simulink model "imcpendel4"  (R2021b)
settings: Solver=daessc  StartTime=0.0  StopTime=100  RelTol=1e-3
values from neighbouring files (symbols this model uses):
  A = eval(A)    [pendulum1.m]
  B = eval(B)    [pendulum1.m]
  C = [1 0]    [pendulum1.m]
  D = [0]    [pendulum1.m]
  G_star_filter = G_star_stable*G_filter    [pendulum1.m]
  xR = [pi; 0]    [pendulum1.m]
settings Model: Creator=mluser  LastModifiedBy=1star
settings DebuggingCC: UnconnectedInputMsg=none  UnconnectedOutputMsg=none  UnconnectedLineMsg=none
settings ModelReferenceCC: EnableRefExpFcnMdlSchedulingChecks=off
settings RTWCC: DLArmComputeVersion=20.02.1

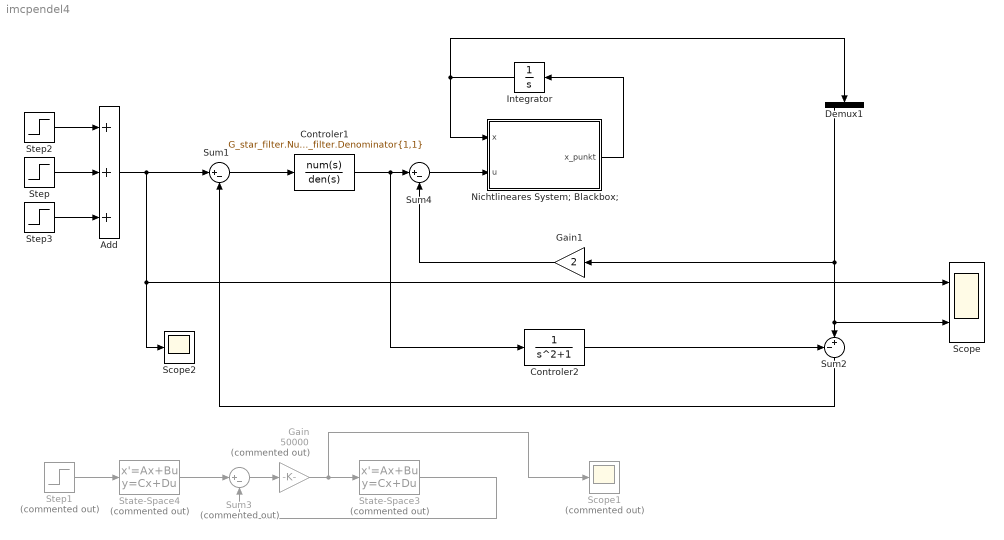
== system imcpendel4 ==
  Add : Sum  Inputs=+++
  Controler1 : TransferFcn  Numerator=G_star_filter.Numerator{1,1}  Denominator=G_star_filter.Denominator{1,1}
  Controler2 : TransferFcn  Numerator=1  Denominator=[1 0 1]
  Demux1 : Demux  Outputs=2
  Gain : Gain  Commented=on  Gain=50000
  Gain1 : Gain  Gain=2
  Integrator : Integrator  InitialCondition=xR
  Nichtlineares System; Blackbox; : MATLAB Function
  Scope : Scope  NumInputPorts=2
  Scope1 : Scope  Commented=on
  Scope2 : Scope
  State-Space3 : StateSpace  Commented=on  A=A  B=B  C=C  D=D  InitialCondition=0
  State-Space4 : StateSpace  Commented=on  A=A  B=B  C=C  D=D  InitialCondition=0
  Step : Step  Time=2  After=0  SampleTime=0
  Step1 : Step  Commented=on  SampleTime=0
  Step2 : Step  Before=pi  After=pi  SampleTime=0
  Step3 : Step  Time=3  After=0  SampleTime=0
  Sum1 : Sum  Inputs=|+-
  Sum2 : Sum  Inputs=-+|
  Sum3 : Sum  Commented=on  Inputs=|+-
  Sum4 : Sum  Inputs=|+-
  wires:
  Controler2/1 -> Sum2/1
  Sum1/1 -> Controler1/1
  State-Space3/1 -> Sum3/2
  Step1/1 -> State-Space4/1
  State-Space4/1 -> Sum3/1
  Gain/1 -> Scope1/1, State-Space3/1
  Sum3/1 -> Gain/1
  Add/1 -> Scope2/1, Scope/1, Sum1/1
  Step/1 -> Add/2
  Step3/1 -> Add/3
  Step2/1 -> Add/1
  Nichtlineares System; Blackbox;/1(x_punkt) -> Integrator/1
  Sum2/1 -> Sum1/2
  Gain1/1 -> Sum4/2
  Controler1/1 -> Controler2/1, Sum4/1
  Sum4/1 -> Nichtlineares System; Blackbox;/2(u)
  Integrator/1 -> Demux1/1, Nichtlineares System; Blackbox;/1(x)
  Demux1/1 -> Sum2/2, Scope/2, Gain1/1

== matlab function imcpendel4/Nichtlineares System; Blackbox; ==
  data: x input; x_punkt output; u input
function x_punkt  = fcn(x, u)
x1_punkt = x(2); 
x2_punkt = -sin(x(1)) + u;

x_punkt = [x1_punkt; x2_punkt];
